simulink model "sl_robreg1_CR_MM_dezPD"  (R2023b)
settings: Solver=ode15s  StartTime=0.0  StopTime=6  RelTol=1e-3
undefined symbols (not defined in the file): C1, C3, C5, C7
libraries: robotmaniplib x1, simulink x1, robotcorelib x1
settings Model: Creator=jaekel  LastModifiedBy=gnamp
settings DataIOCC: InspectSignalLogs=on

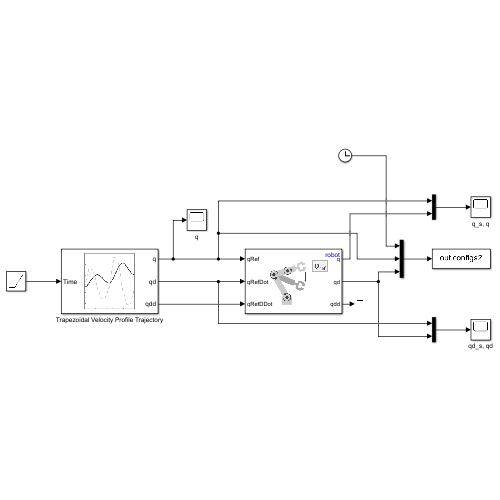
[thumbnail: Simulink's stored preview of the top-level diagram]
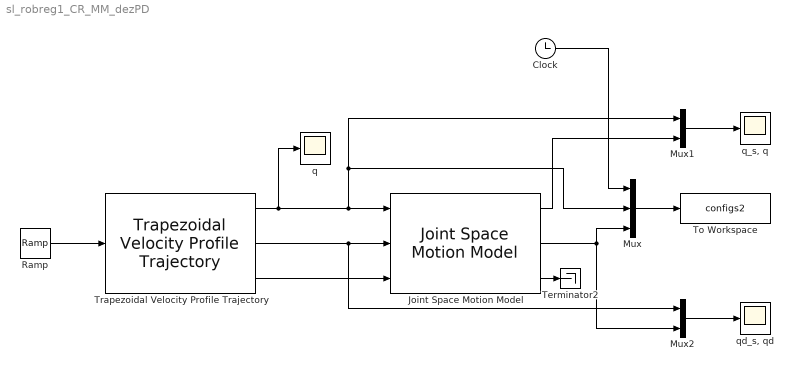
== system sl_robreg1_CR_MM_dezPD ==
  Clock : Clock
  Joint Space Motion Model : robotmaniplib/Joint Space Motion Model  RigidBodyTree=robot  MotionType=Independent Joint Motion  ProportionalGain=100  DerivativeGain=10  ErrorDynamicsSpecification=Step Response  DampingRatio=0.59116  NaturalFrequency=6.7664  SettlingTime=1  Overshoot=0.1  ShowExternalForcePort=off  InitConfig=C1'  InitJointVel=0  SimulateUsing=Interpreted execution
  Mux : Mux  Inputs=3
  Mux1 : Mux  Inputs=2
  Mux2 : Mux  Inputs=2
  Ramp : simulink/Sources/Ramp  slope=1  start=0  InitialOutput=0
  Terminator2 : Terminator
  To Workspace : ToWorkspace  VariableName=configs2  SampleTime=-1
  Trapezoidal Velocity Profile Trajectory : robotcorelib/Trapezoidal Velocity Profile Trajectory  WaypointSource=Internal  Waypoints=[,C1',C2',C3',C4',C5',C6',C7']  NumParams=1  Parameter1=End Time  Parameter2=End Time  ParameterSource=Internal  PeakVelocity=[ 2; 2 ]  Acceleration=[ 1; 2 ]  EndTime=1  AccelTime=[ 1; 2 ]  SimulateUsing=Interpreted execution
  q : Scope
  "q_s, q" : Scope
  "qd_s, qd" : Scope
  wires:
  Trapezoidal Velocity Profile Trajectory/1 -> q/1, Mux/2, Mux1/1, Joint Space Motion Model/1
  Trapezoidal Velocity Profile Trajectory/2 -> Mux2/1, Joint Space Motion Model/2
  Ramp/1 -> Trapezoidal Velocity Profile Trajectory/1
  Mux1/1 -> "q_s, q"/1
  Mux/1 -> To Workspace/1
  Joint Space Motion Model/1 -> Mux1/2
  Clock/1 -> Mux/1
  Joint Space Motion Model/2 -> Mux/3, Mux2/2
  Mux2/1 -> "qd_s, qd"/1
  Joint Space Motion Model/3 -> Terminator2/1
  Trapezoidal Velocity Profile Trajectory/3 -> Joint Space Motion Model/3
